simulink model "main_sim_adapt_Gref_SP"  (Simulink 7.2)
settings: Solver=ode2  SolverMode=SingleTasking  StartTime=0.0  StopTime=tsim_max  FixedStep=dtsim  RelTol=1e-3
StopFcn:
  | %mkplt
values from neighbouring files (symbols this model uses):
  aero_surf_qbar_off = get_value('aero_surf_qbar_off')    [setup_claw.m]
  aero_surf_qbar_on = get_value('aero_surf_qbar_on')    [setup_claw.m]
  assertion_time = get_value('assertion_time')    [setup_sim.m]
  att_cmd_select = get_value('att_cmd_select')    [setup_sim.m]
  att_trim_IC = orientation.att'    [setup_claw.m]
  att_type_numbers = cell2mat(struct2cell(att_type))    [setup_constants.m]
  chi_trim_IC = orientation.Vchigam(2)    [setup_claw.m]
  command_time = engage_time + 2.0    [setup_sim.m]
  compute_all_rate_cols = get_value('compute_all_rate_cols')    [setup_claw.m]
  compute_all_vel_cols = get_value('compute_all_vel_cols')    [setup_claw.m]
  da_trim_IC = tmp(1)    [setup_claw.m]
  dc_L2W_IC = orientation.dc_L2W    [setup_claw.m]
  de_trim_IC = tmp(2)    [setup_claw.m]
  dr_trim_IC = tmp(3)    [setup_claw.m]
  dtsim = get_value('dtsim')    [setup_sim.m]
  E_trim_IC = MACH_pos_IC(2)    [setup_claw.m]
  Ed_trim_IC = MACH_vel_IC(2)    [setup_claw.m]
  gain_set = gain_set_next    (= 1)    [setup_claw.m]
  gain_var_struct = rmfield(gain_var_struct,setdiff(fieldnames(gain_var_struct),{'name','size'}))    [setup_claw.m]
  gamma_trim_IC = orientation.Vchigam(3)    [setup_claw.m]
  h_trim_IC = MACH_pos_IC(3)    [setup_claw.m]
  hd_trim_IC = MACH_vel_IC(3)    [setup_claw.m]
  ideal_vel_Kb = MACH_vel_Kb(1)    [setup_sim.m]
  MACH = rmfield(MACH,'vel_throt_lrlim')    [setup_claw.m]
  MACH_att_fb = get_value('MACH_att_fb','onerror',0)    [setup_claw.m]
  MACH_att_int_IC = (1-MACH_att_Kc).*MACH_quat_IC'    [setup_ideal.m]
  MACH_att_Kb = repval(att_kbnom,MACH.att_num_cv)    [setup_claw.m]
  MACH_att_Kc = Ki2Kc(MACH_att_Ki)    [setup_ideal.m]
  MACH_att_Ki = repval(att_fi,MACH.att_num_cv)    [setup_claw.m]
  MACH_gain_mat = vertcat(MACH_gain_mat, this_gain_mat)    [setup_claw.m]
  MACH_mass_IC = obac_params.mass_IC    [setup_claw.m]
  MACH_pos_IC = x_obac_IC(MACH.NEh_idx)    [setup_claw.m]
  MACH_pos_int_IC = (1-MACH_pos_Kc).*MACH_pos_IC' + MACH_vel_IC'./MACH_pos_Kb    [setup_ideal.m]
  MACH_pos_Kb = repval(pos_kbnom,MACH.pos_num_cv)    [setup_claw.m]
  MACH_pos_Kc = Ki2Kc(MACH_pos_Ki)    [setup_ideal.m]
  MACH_pos_Ki = repval(pos_fi,MACH.pos_num_cv)    [setup_claw.m]
  MACH_pqr_Bmat_IC = Bo(MACH.pqr_idx,MACH.pqr_u_idx)    [setup_claw.m]
  MACH_pqr_IC = pqr_trim_IC    [setup_claw.m]
  MACH_pqr_int_IC = (1-MACH_pqr_Kc).*MACH_pqr_IC'    [setup_ideal.m]
  MACH_pqr_Kb = repval(pqr_kbnom,MACH.pqr_num_cv)    [setup_claw.m]
  MACH_pqr_Kc = Ki2Kc(MACH_pqr_Ki)    [setup_ideal.m]
  MACH_pqr_Ki = repval(pqr_fi,MACH.pqr_num_cv)    [setup_claw.m]
  MACH_pqr_u_IC = [ vanes_trim_IC; tvc_trim_IC; rcs_trim_IC ]    [setup_claw.m]
  MACH_quat_IC = quat_trim_IC    [setup_claw.m]
  MACH_throttle_IC = throttle_trim_IC    [setup_claw.m]
  MACH_U_nom_IC = zeros(MACH.num_u,1)    [setup_claw.m]
  MACH_vel_Bmat_IC = MACH_vel_Bmat_IC*inv(vel_perts)    [setup_claw.m]
  MACH_vel_cvdnom_IC = repval(get_value('vel_cvdnom_IC','onerror',MACH_vel_cvdnom_IC),length(MACH_vel_cvdnom_IC))'    [setup_claw.m]
  MACH_vel_IC = orientation.NdEdhd'    [setup_claw.m]
  MACH_vel_int_IC = (1-MACH_vel_Kc).*MACH_vel_IC'    [setup_ideal.m]
  MACH_vel_Kb = repval(vel_kbnom,MACH.vel_num_cv)    [setup_claw.m]
  MACH_vel_Kc = Ki2Kc(MACH_vel_Ki)    [setup_ideal.m]
  MACH_vel_Ki = repval(vel_fi,MACH.vel_num_cv)    [setup_claw.m]
  MACH_vel_uold_IC = [ MACH_quat_IC; MACH_throttle_IC ]    [setup_claw.m]
  N_trim_IC = MACH_pos_IC(1)    [setup_claw.m]
  Nd_trim_IC = MACH_vel_IC(1)    [setup_claw.m]
  obac_params = define_model('obac', get_value('obac_model_type'))    [setup_claw.m]
  pos_cmd_select = get_value('pos_cmd_select')    [setup_sim.m]
  pqr_trim_IC = [ 0 0 0 ]'    [setup_claw.m]
  rate_cmd_select = get_value('rate_cmd_select')    [setup_sim.m]
  rcs_cvddes_thresh = get_value('rcs_cvddes_thresh')    [setup_claw.m]
  reset_camcmd_on_entry = get_value('reset_camcmd_on_entry')    [setup_claw.m]
  throttle_trim_IC = u_obac_IC(MACH.throttle_idx)    [setup_claw.m]
  trac_params = define_model('trac', get_value('trac_model_type','onerror',obac_params.model_type))    [setup_sim.m]
  use_auto_att_type = get_value('use_auto_att_type','onerror',0)    [setup_claw.m]
  use_eow_as_iv = get_value('use_eow_as_iv')    [setup_claw.m]
  use_full_surf_cmd = get_value('use_full_surf_cmd')    [setup_sim.m]
  use_nav = get_value('use_nav')    [setup_claw.m]
  use_NdEdh_pos = get_value('use_NdEdh_pos')    [setup_claw.m]
  use_pos_fltpath_lim = get_value('use_pos_fltpath_lim')    [setup_claw.m]
  use_throt_estimate = get_value('use_throt_estimate')    [setup_claw.m]
  use_variable_mass = get_value('use_variable_mass')    [setup_claw.m]
  use_wind_est = get_value('use_wind_est')    [setup_claw.m]
  V_trim_IC = orientation.Vchigam(1)    [setup_claw.m]
  vel_cmd_ramp_time = get_value('vel_cmd_ramp_time')    [setup_claw.m]
  vel_cmd_select = get_value('vel_cmd_select')    [setup_sim.m]
  x_trac_IC = x_obac_IC    [setup_sim.m]
undefined symbols (not defined in the file or in its folder): accel_cmd, alpha_trim, Am, att_type, B1, bb_ellipsoid, bb_params, Bm, C, constants, cosA, DiscIntNeverNeededParam, DZkx, DZtheta, E_rwy, Ed_cmd, eow_boundary, flag_autoadapt, flag_exsig, flag_uad, full_surf_llim, full_surf_ulim, gam_cmd_descent, gam_cmd_preflare, gamdot_cmd_descent, gamdot_cmd_flare, gamdot_cmd_preflare, Gamtheta, Gamx, hd_cmd, in_error_thresh, in_exsig_vecin, in_exsig_vecout, in_reset_stoptime, in_t_exsig, in_t_timer, in_tadaptoff_forced, in_tadapton_forced, Kb, Kxhat0, Kxnom, Kxstar, max_chi_cmd, max_LOS_rate, max_vel_cmd, min_chi_cmd, min_vel_cmd, modes, N_rwy, Nd_cmd, Nrbf, P, pos, Sig, sinA, target_pos_IC, target_range_blind, target_range_detect, target_range_homing, target_vel_IC ... (+11)
libraries: simulink x44, utility_lib x36, mach_lib x24, model_lib x13, simulink_need_slupdate x8, models x8
(part 2 of 8)

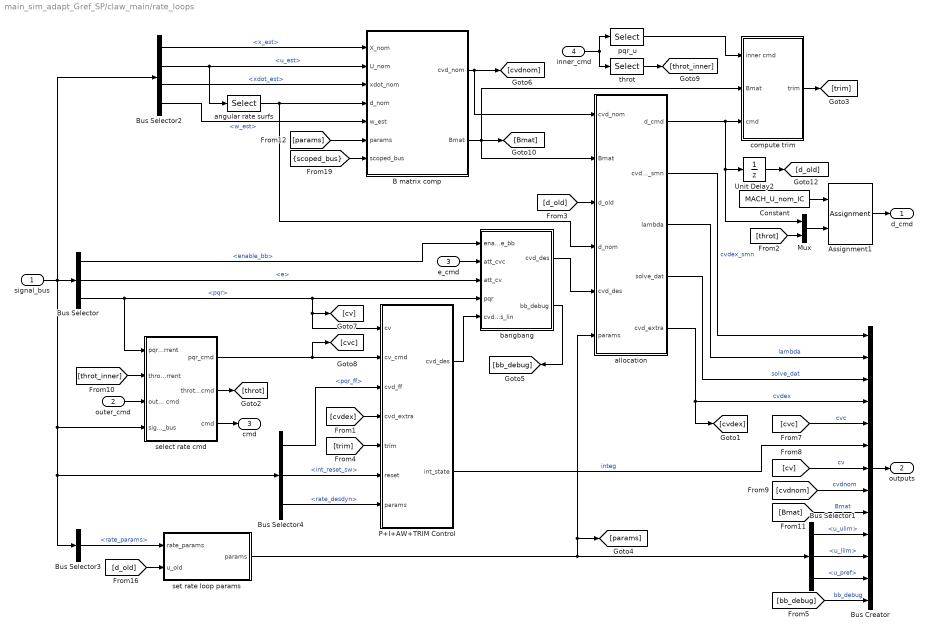
== system main_sim_adapt_Gref_SP/claw_main/rate_loops ==
  signal_bus : Inport  OutDataType=sfix(16)  OutScaling=2^0
  outer_cmd : Inport  Port=2  OutDataType=sfix(16)  OutScaling=2^0
  e_cmd : Inport  Port=3  OutDataType=sfix(16)  OutScaling=2^0
  inner_cmd : Inport  Port=4  OutDataType=sfix(16)  OutScaling=2^0
  Assignment1 : Assignment  IndexOptions=Index vector (dialog)  Indices=[MACH.pqr_u_idx MACH.throttle_idx]  OutputSizes=[1 1]
  B matrix comp : Subsystem  TreatAsAtomicUnit=on
  Bus Creator : BusCreator  Inputs=13
  Bus Selector : BusSelector  OutputSignals=control_params.enable_bb,x_est.e,x_est.pqr
  Bus Selector1 : BusSelector  OutputSignals=u_ulim,u_llim,u_pref
  Bus Selector2 : BusSelector  OutputSignals=x_est,u_est,xdot_est,y_meas.w_est
  Bus Selector3 : BusSelector  OutputSignals=control_params.rate_params
  Bus Selector4 : BusSelector  OutputSignals=feed_forward.pqr_ff,mode_sw.int_reset_sw,control_params.rate_desdyn
  Constant : Constant  Value=MACH_U_nom_IC  OutDataType=sfix(16)  OutScaling=2^0
  Mux : Mux  Inputs=2
  P+I+AW+TRIM Control : Subsystem  AncestorBlock=mach_lib/P+I+AW+TRIM Control
  Unit Delay2 : UnitDelay  X0=MACH_pqr_u_IC  SampleTime=-1
  allocation : Subsystem
  angular rate surfs : Selector  InputPortWidth=MACH.num_u  IndexOptions=Index vector (dialog)  Indices=MACH.pqr_u_idx  OutputSizes=1
  bangbang : Subsystem
  compute trim : Subsystem
  pqr_u : Selector  InputPortWidth=MACH.num_u  IndexOptions=Index vector (dialog)  Indices=MACH.pqr_u_idx  OutputSizes=1
  select rate cmd : Subsystem
  set rate loop params : Subsystem
  throt : Selector  InputPortWidth=MACH.num_u  IndexOptions=Index vector (dialog)  Indices=MACH.throttle_idx  OutputSizes=1
  d_cmd : Outport  OutDataType=sfix(16)  OutScaling=2^0
  outputs : Outport  Port=2  OutDataType=sfix(16)  OutScaling=2^0
  cmd : Outport  Port=3  OutDataType=sfix(16)  OutScaling=2^0
  wires:
  angular rate surfs/1 -> B matrix comp/4(d_nom), allocation/4(d_nom)
  outer_cmd/1 -> select rate cmd/3(outer cmd)
  B matrix comp/1(cvd_nom) -> [cvdnom], allocation/1(cvd_nom)
  P+I+AW+TRIM Control/2(int_state) -> Bus Creator/6  "integ"
  signal_bus/1 -> Bus Selector2/1, Bus Selector/1, Bus Selector3/1, Bus Selector4/1, select rate cmd/4(signal_bus)
  compute trim/1(trim) -> [trim]
  inner_cmd/1 -> pqr_u/1, throt/1
  select rate cmd/2(throt_cmd) -> [throt]
  select rate cmd/1(pqr_cmd) -> [cvc], P+I+AW+TRIM Control/2(cv_cmd)
  [throt_inner] -> select rate cmd/2(throt_current)
  [cvc] -> Bus Creator/5  "cvc"
  [cv] -> Bus Creator/7  "cv"
  [cvdnom] -> Bus Creator/8  "cvdnom"
  set rate loop params/1(params) -> Bus Selector1/1, allocation/6(params), [params]
  Assignment1/1 -> d_cmd/1
  throt/1 -> [throt_inner]
  [trim] -> P+I+AW+TRIM Control/5(trim)
  [cvdex] -> P+I+AW+TRIM Control/4(cvd_extra)
  Bus Selector/3 -> select rate cmd/1(pqr_current), bangbang/4(pqr), P+I+AW+TRIM Control/1(cv), [cv]  "<pqr>"
  Bus Selector4/1 -> P+I+AW+TRIM Control/3(cvd_ff)  "<pqr_ff>"
  Bus Selector4/2 -> P+I+AW+TRIM Control/6(reset)  "<int_reset_sw>"
  [Bmat] -> Bus Creator/9  "Bmat"
  Bus Selector1/1 -> Bus Creator/10  "<u_ulim>"
  Bus Selector1/2 -> Bus Creator/11  "<u_llim>"
  [d_old] -> set rate loop params/2(u_old)
  pqr_u/1 -> compute trim/1(inner cmd)
  Constant/1 -> Assignment1/1
  Mux/1 -> Assignment1/2
  Bus Selector2/1 -> B matrix comp/1(X_nom)  "<x_est>"
  Bus Selector2/2 -> angular rate surfs/1, B matrix comp/2(U_nom)  "<u_est>"
  Bus Selector2/3 -> B matrix comp/3(xdot_nom)  "<xdot_est>"
  Bus Selector2/4 -> B matrix comp/5(w_est)  "<w_est>"
  Bus Selector1/3 -> Bus Creator/12  "<u_pref>"
  allocation/5(cvd_extra) -> Bus Creator/4, [cvdex]  "cvdex"
  [throt] -> Mux/2
  Unit Delay2/1 -> [d_old]
  allocation/1(d_cmd) -> compute trim/3(cmd), Mux/1, Unit Delay2/1
  [d_old] -> allocation/3(d_old)
  B matrix comp/2(Bmat) -> compute trim/2(Bmat), [Bmat], allocation/2(Bmat)
  allocation/3(lambda) -> Bus Creator/2  "lambda"
  allocation/4(solve_dat) -> Bus Creator/3  "solve_dat"
  Bus Creator/1 -> outputs/1
  [scoped_bus] -> B matrix comp/7(scoped_bus)
  [params] -> B matrix comp/6(params)
  Bus Selector4/3 -> P+I+AW+TRIM Control/7(params)  "<rate_desdyn>"
  allocation/2(cvd_extra_smn) -> Bus Creator/1  "cvdex_smn"
  bangbang/1(cvd_des) -> allocation/5(cvd_des)
  e_cmd/1 -> bangbang/2(att_cvc)
  Bus Selector/2 -> bangbang/3(att_cv)  "<e>"
  P+I+AW+TRIM Control/1(cvd_des) -> bangbang/5(cvd_des_lin)
  Bus Selector/1 -> bangbang/1(enable_bb)  "<enable_bb>"
  bangbang/2(bb_debug) -> [bb_debug]
  [bb_debug] -> Bus Creator/13  "bb_debug"
  select rate cmd/3(cmd) -> cmd/1
  Bus Selector3/1 -> set rate loop params/1(rate_params)  "<rate_params>"

== system main_sim_adapt_Gref_SP/claw_main/servo commands  when not engaged ==
  note: for OAV/MAV during "pre-takeoff",
      |  the rate inner_cmd throt was set to takeoff throt
      | to allow integrators to trim for anticipated takeoff.
      | This should be revisited within current CLAW
      | before being used again.
  signal_bus : Inport  OutDataType=sfix(16)  OutScaling=2^0
  outer_cmd : Inport  Port=2  OutDataType=sfix(16)  OutScaling=2^0
  Bus Selector1 : BusSelector  OutputSignals=mode_sw.pre_takeoff_sw,mode_sw.engaged_sw,mode_sw.full_surf_cmd_sw,cmd_bus.autopilot_cmd,full_surf.full_surf_cmd
  Constant1 : Constant  Value=MACH.pre_takeoff_u_backtrim  OutDataType=sfix(16)  OutScaling=2^0
  Multiport Switch : MultiPortSwitch  Inputs=2  zeroidx=on
  Multiport Switch1 : MultiPortSwitch  Inputs=2  zeroidx=on
  Multiport Switch2 : MultiPortSwitch  Inputs=2  zeroidx=on
  pseudo surf cmd : Subsystem
  u_out : Outport  OutDataType=sfix(16)  OutScaling=2^0
  u_backtrim : Outport  Port=2  OutDataType=sfix(16)  OutScaling=2^0
  wires:
  signal_bus/1 -> Bus Selector1/1
  Bus Selector1/1 -> Multiport Switch/1  "<pre_takeoff_sw>"
  Multiport Switch1/1 -> Multiport Switch/2, u_out/1
  Constant1/1 -> Multiport Switch/3
  Bus Selector1/2 -> Multiport Switch1/1  "<engaged_sw>"
  Bus Selector1/3 -> Multiport Switch2/1  "<full_surf_cmd_sw>"
  Bus Selector1/4 -> pseudo surf cmd/1(autopilot_cmd)  "<autopilot_cmd>"
  pseudo surf cmd/1(surf_cmd) -> Multiport Switch2/2
  Bus Selector1/5 -> Multiport Switch2/3  "<full_surf_cmd>"
  Multiport Switch2/1 -> Multiport Switch1/2
  outer_cmd/1 -> Multiport Switch1/3
  Multiport Switch/1 -> u_backtrim/1

== system main_sim_adapt_Gref_SP/claw_main/set scoped signals ==
  signal_bus : Inport  OutDataType=sfix(16)  OutScaling=2^0
  Bus Selector3 : BusSelector  OutputSignals=y_meas.h_geodetic,mode_sw.use_held_aero_obac_sw,y_meas.w_est,y_meas.NEh_dot,mode_sw.att_type,u_est,engines
  Gain1 : Gain  Orientation=left  Gain=use_variable_mass  ParameterDataType=sfix(16)  ParameterScaling=2^0  OutDataType=sfix(16)  OutScaling=2^0
  hold altitude : model_lib/hold input  SystemSampleTime=-1
  mass : DiscreteIntegrator  gainval=1  InitialCondition=MACH_mass_IC  SampleTime=-1  OutDataType=sfix(16)  OutScaling=2^0  ICPrevOutput=DiscIntNeverNeededParam  ICPrevScaledInput=DiscIntNeverNeededParam
  set scoped bus : model_lib/set scoped bus  SystemSampleTime=-1  vehicle_params=obac_params
  set scoped signals : model_lib/set scoped signals  SystemSampleTime=-1
  scoped_bus : Outport  OutDataType=sfix(16)  OutScaling=2^0
  wires:
  signal_bus/1 -> Bus Selector3/1
  Gain1/1 -> mass/1
  Bus Selector3/1 -> hold altitude/1  "<h_geodetic>"
  set scoped bus/2 -> Gain1/1
  set scoped bus/1 -> set scoped signals/1, scoped_bus/1
  mass/1 -> set scoped bus/7
  Bus Selector3/2 -> hold altitude/2  "<use_held_aero_obac_sw>"
  hold altitude/1 -> set scoped bus/1
  Bus Selector3/3 -> set scoped bus/2  "<w_est>"
  Bus Selector3/4 -> set scoped bus/3  "<NEh_dot>"
  Bus Selector3/5 -> set scoped bus/4  "<att_type>"
  Bus Selector3/6 -> set scoped bus/5  "<u_est>"
  Bus Selector3/7 -> set scoped bus/6  "<engines>"

== system main_sim_adapt_Gref_SP/claw_main/state est ==
  u_old : Inport  OutDataType=sfix(16)  OutScaling=2^0
  sensors : Inport  Port=2  OutDataType=sfix(16)  OutScaling=2^0
  signal_bus : Inport  Port=3  OutDataType=sfix(16)  OutScaling=2^0
  Bus Creator : BusCreator  Inputs=12
  Bus Creator1 : BusCreator  Inputs=6
  Bus Selector : BusSelector  OutputSignals=mode_sw.reset_pos_sw,mode_sw.nav_enable_sw,mode_sw.wind_est_sw
  Bus Selector1 : BusSelector  OutputSignals=nav_ok,pqr,NED_dot,latlonh,e
  Bus Selector2 : BusSelector  OutputSignals=aero_env.Mach,aero_env.vel,aero_env.alpha,aero_env.beta,aero_env.uvw_rw,aero_env.qbar
  Bus Selector3 : BusSelector  OutputSignals=u_meas,seeker,accels_cg
  Logical Operator : Logic  AllPortsSameDT=off  OutDataTypeMode=boolean  OutDataTypeStr=boolean
  beta_360 : Fcn  Expr=atan2(u(2),u(1))
  cl model : models/gtm-obac  SystemSampleTime=-1
  process inputs : Subsystem
  process sensors : Subsystem
  wind estimator : Subsystem
  y_meas : Outport  OutDataType=sfix(16)  OutScaling=2^0
  x_est : Outport  Port=2  OutDataType=sfix(16)  OutScaling=2^0
  xdot_est : Outport  Port=3  OutDataType=sfix(16)  OutScaling=2^0
  u_est : Outport  Port=4  OutDataType=sfix(16)  OutScaling=2^0
  aero_env_est : Outport  Port=5  OutDataType=sfix(16)  OutScaling=2^0
  w_est_debug : Outport  Port=6  OutDataType=sfix(16)  OutScaling=2^0
  wires:
  sensors/1 -> Bus Selector3/1, process inputs/2(sensors), wind estimator/3(sensors), Bus Selector1/1
  wind estimator/1(w_est) -> cl model/3, Bus Creator/12  "w_est"
  process sensors/8(dircos) -> wind estimator/1(dircos), Bus Creator/11  "dircos"
  cl model/1 -> xdot_est/1
  process sensors/9(x_est) -> cl model/1, wind estimator/2(x), x_est/1
  signal_bus/1 -> Bus Selector/1
  Bus Selector/1 -> process sensors/1(reset_pos)  "<reset_pos_sw>"
  Bus Selector/3 -> wind estimator/5(wind_est_sw)  "<wind_est_sw>"
  process inputs/1(u_est) -> u_est/1, cl model/2, wind estimator/4(u)
  Bus Selector1/2 -> process sensors/3(pqr)  "<pqr>"
  Bus Selector1/3 -> process sensors/4(NED_dot)  "<NED_dot>"
  Bus Selector1/4 -> process sensors/5(latlonh)  "<latlonh>"
  Bus Selector1/5 -> process sensors/6(e)  "<e>"
  process sensors/2(h_geodetic) -> Bus Creator/5  "h_geodetic"
  process sensors/3(NEh_nav) -> Bus Creator/6  "NEh_nav"
  process sensors/4(nav_valid) -> Bus Creator/7  "nav_valid"
  process sensors/5(NEh_dot) -> Bus Creator/8  "NEh_dot"
  process sensors/1(vehicle_origin) -> Bus Creator/4  "vehicle_origin"
  process sensors/7(cvc_origin) -> Bus Creator/10  "cvc_origin"
  u_old/1 -> process inputs/1(u_old)
  wind estimator/2(w_est_debug) -> w_est_debug/1
  cl model/2 -> Bus Selector2/1
  Bus Creator1/1 -> aero_env_est/1
  Logical Operator/1 -> process sensors/2(nav_ok)
  Bus Selector1/1 -> Logical Operator/2  "<nav_ok>"
  Bus Selector/2 -> Logical Operator/1  "<nav_enable_sw>"
  Bus Selector2/5 -> beta_360/1  "<uvw_rw>"
  process sensors/6(dc_fltpath) -> Bus Creator/9  "dc_fltpath"
  beta_360/1 -> Bus Creator1/5  "beta_360"
  Bus Selector2/1 -> Bus Creator1/1  "<Mach>"
  Bus Selector2/2 -> Bus Creator1/2  "<vel>"
  Bus Selector2/3 -> Bus Creator1/3  "<alpha>"
  Bus Selector2/4 -> Bus Creator1/4  "<beta>"
  Bus Selector2/6 -> Bus Creator1/6  "<qbar>"
  Bus Selector3/1 -> Bus Creator/1  "<u_meas>"
  Bus Selector3/2 -> Bus Creator/2  "<seeker>"
  Bus Selector3/3 -> Bus Creator/3  "<accels_cg>"
  Bus Creator/1 -> y_meas/1

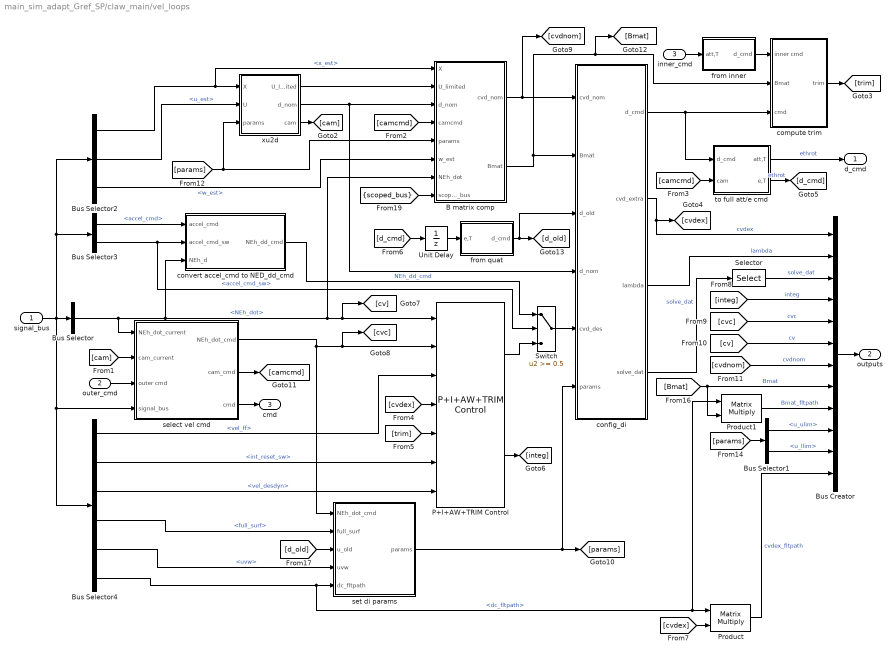
== system main_sim_adapt_Gref_SP/claw_main/vel_loops ==
  signal_bus : Inport  OutDataType=sfix(16)  OutScaling=2^0
  outer_cmd : Inport  Port=2  OutDataType=sfix(16)  OutScaling=2^0
  inner_cmd : Inport  Port=3  OutDataType=sfix(16)  OutScaling=2^0
  B matrix comp : Subsystem
  Bus Creator : BusCreator  Inputs=12
  Bus Selector : BusSelector  OutputSignals=y_meas.NEh_dot
  Bus Selector1 : BusSelector  OutputSignals=u_ulim,u_llim
  Bus Selector2 : BusSelector  OutputSignals=x_est,u_est,y_meas.w_est
  Bus Selector3 : BusSelector  OutputSignals=control_params.accel_cmd,control_params.accel_cmd_sw
  Bus Selector4 : BusSelector  OutputSignals=feed_forward.vel_ff,mode_sw.int_reset_sw,control_params.vel_desdyn,full_surf,x_est.uvw,y_meas.dc_fltpath
  P+I+AW+TRIM Control : mach_lib/P+I+AW+TRIM Control  SystemSampleTime=-1
  Product : Product  Multiplication=Matrix(*)  OutDataType=sfix(16)  OutScaling=2^0  RndMeth=Zero
  Product1 : Product  Multiplication=Matrix(*)  OutDataType=sfix(16)  OutScaling=2^0  RndMeth=Zero
  Selector : Selector  NumberOfDimensions=2  InputPortWidth=MACH.num_u  IndexOptions=Index vector (dialog),Index vector (dialog)  Indices=1:9,1:2  OutputSizes=1
  Switch : Switch  Threshold=0.5
  Unit Delay : UnitDelay  X0=MACH_vel_uold_IC  SampleTime=-1
  compute trim : Subsystem
  config_di : Subsystem  BlockChoice=di_smn  mask{num_cv=MACH.vel_num_cv, num_u=MACH.vel_num_u, wght_cv_type=MACH.vel_wght_cv_type}
      link override di_smn/config_smn/smn_sfunc: sfunc_name=MACH.smn_sfunc_name
      link override di_smn/config_smn/smn_sfunc/S-Function: FunctionName=smn_sfunc_gam_mpass_epsposdef
      settings: AttributesFormatString=%<BlockChoice>  TemplateBlock=mach_lib/config_di  MemberBlocks=di_pseudoinv,di_smn
  convert accel_cmd to NED_dd_cmd : Subsystem  TreatAsAtomicUnit=on
  from inner : Subsystem
  from quat : Subsystem
  select vel cmd : Subsystem
  set di params : Subsystem
  to full att/e cmd : Subsystem
  xu2d : Subsystem
  d_cmd : Outport  OutDataType=sfix(16)  OutScaling=2^0
  outputs : Outport  Port=2  OutDataType=sfix(16)  OutScaling=2^0
  cmd : Outport  Port=3  OutDataType=sfix(16)  OutScaling=2^0
  wires:
  B matrix comp/2(Bmat) -> config_di/2(Bmat), compute trim/2(Bmat), [Bmat]
  to full att/e cmd/1(att,T) -> d_cmd/1  "ethrot"
  config_di/1(d_cmd) -> compute trim/3(cmd), to full att/e cmd/1(d_cmd)
  P+I+AW+TRIM Control/2 -> [integ]
  xu2d/2(d_nom) -> config_di/4(d_nom), B matrix comp/3(d_nom)
  Bus Selector/1 -> convert accel_cmd to NED_dd_cmd/3(NEh_d), B matrix comp/7(NEh_dot), P+I+AW+TRIM Control/1, [cv], select vel cmd/1(NEh_dot_current)  "<NEh_dot>"
  xu2d/3(cam) -> [cam]
  [cam] -> select vel cmd/2(cam_current)
  compute trim/1(trim) -> [trim]
  inner_cmd/1 -> from inner/1(att,T)
  from inner/1(d_cmd) -> compute trim/1(inner cmd)
  [camcmd] -> to full att/e cmd/2(cam)
  Bus Selector2/3 -> B matrix comp/6(w_est)  "<w_est>"
  [d_cmd] -> Unit Delay/1
  Unit Delay/1 -> from quat/1(e,T)
  set di params/1(params) -> [params], config_di/6(params)
  [params] -> xu2d/3(params), B matrix comp/5(params)
  xu2d/1(U_limited) -> B matrix comp/2(U_limited)
  [integ] -> Bus Creator/4  "integ"
  [cvc] -> Bus Creator/5  "cvc"
  [cv] -> Bus Creator/6  "cv"
  [cvdnom] -> Bus Creator/7  "cvdnom"
  [trim] -> P+I+AW+TRIM Control/5
  [cvdex] -> P+I+AW+TRIM Control/4
  Bus Selector4/2 -> P+I+AW+TRIM Control/6  "<int_reset_sw>"
  Bus Selector4/1 -> P+I+AW+TRIM Control/3  "<vel_ff>"
  B matrix comp/1(cvd_nom) -> [cvdnom], config_di/1(cvd_nom)
  [Bmat] -> Product1/2, Bus Creator/8  "Bmat"
  config_di/2(cvd_extra) -> [cvdex], Bus Creator/1  "cvdex"
  from quat/1(d_cmd) -> [d_old], config_di/3(d_old)
  Bus Selector4/4 -> set di params/2(full_surf)  "<full_surf>"
  Product/1 -> Bus Creator/12  "cvdex_fltpath"
  [params] -> Bus Selector1/1
  Bus Selector1/1 -> Bus Creator/10  "<u_ulim>"
  Bus Selector1/2 -> Bus Creator/11  "<u_llim>"
  [d_old] -> set di params/3(u_old)
  Bus Selector4/5 -> set di params/4(uvw)  "<uvw>"
  config_di/3(lambda) -> Bus Creator/2  "lambda"
  config_di/4(solve_dat) -> Selector/1  "solve_dat"
  [cvdex] -> Product/2
  Selector/1 -> Bus Creator/3  "solve_dat"
  [camcmd] -> B matrix comp/4(camcmd)
  [scoped_bus] -> B matrix comp/8(scoped_bus)
  Bus Selector2/1 -> xu2d/1(X), B matrix comp/1(X)  "<x_est>"
  Bus Selector2/2 -> xu2d/2(U)  "<u_est>"
  Bus Selector4/3 -> P+I+AW+TRIM Control/7  "<vel_desdyn>"
  Bus Selector3/1 -> convert accel_cmd to NED_dd_cmd/1(accel_cmd)  "<accel_cmd>"
  Switch/1 -> config_di/5(cvd_des)
  P+I+AW+TRIM Control/1 -> Switch/3
  convert accel_cmd to NED_dd_cmd/1(NEh_dd_cmd) -> Switch/1  "NEh_dd_cmd"
  signal_bus/1 -> Bus Selector/1, Bus Selector3/1, Bus Selector2/1, Bus Selector4/1, select vel cmd/4(signal_bus)
  Bus Selector3/2 -> convert accel_cmd to NED_dd_cmd/2(accel_cmd_sw), Switch/2  "<accel_cmd_sw>"
  Product1/1 -> Bus Creator/9  "Bmat_fltpath"
  Bus Selector4/6 -> Product/1, Product1/1, set di params/5(dc_fltpath)  "<dc_fltpath>"
  to full att/e cmd/2(e,T) -> [d_cmd]  "ethrot"
  outer_cmd/1 -> select vel cmd/3(outer cmd)
  select vel cmd/3(cmd) -> cmd/1
  select vel cmd/2(cam_cmd) -> [camcmd]
  select vel cmd/1(NEh_dot_cmd) -> set di params/1(NEh_dot_cmd), P+I+AW+TRIM Control/2, [cvc]
  Bus Creator/1 -> outputs/1

== system main_sim_adapt_Gref_SP/control input (modified)/Add Excitation ==
  In : Inport
  Adapt On-Off : Inport  Port=2
  Bus Selector1 : BusSelector  OutputSignals=command
  CMD : Scope
      settings: TimeRange=25  YMin=0  YMax=2  SaveName=ScopeData20
  CMD + EXC : Scope
      settings: TimeRange=25  YMin=-1  YMax=15  SaveName=ScopeData8
  Demux : Demux  Outputs=[1 1 1 1]
  EXC : Scope
      settings: TimeRange=25  YMin=-2  YMax=2  SaveName=ScopeData23
  Excitation  Signal : Subsystem
  Gain1 : Gain  Gain=180/pi  ParameterDataType=sfix(16)  ParameterScaling=2^0  OutDataType=sfix(16)  OutScaling=2^0
  Gain2 : Gain  Gain=180/pi  ParameterDataType=sfix(16)  ParameterScaling=2^0  OutDataType=sfix(16)  OutScaling=2^0
  Gain3 : Gain  Gain=180/pi  ParameterDataType=sfix(16)  ParameterScaling=2^0  OutDataType=sfix(16)  OutScaling=2^0
  Mux : Mux
  Step : Step  Time=in_t_exsig  SampleTime=MACH.dt
  Sum : Sum  Inputs=|++  OutDataType=sfix(16)  OutScaling=2^0
  Terminator : Terminator
  Unit Delay : UnitDelay  SampleTime=MACH.dt
  Out : Outport
  wires:
  Mux/1 -> Out/1
  In/1 -> Bus Selector1/1
  Demux/4 -> Mux/4
  Excitation  Signal/1(exsig) -> Sum/2, Gain3/1
  Sum/1 -> Mux/2, Gain2/1
  Demux/2 -> Sum/1, Gain1/1
  Demux/3 -> Mux/3
  Demux/1 -> Mux/1
  Bus Selector1/1 -> Demux/1  "<command>"
  Gain2/1 -> CMD + EXC/1
  Gain1/1 -> CMD/1
  Gain3/1 -> EXC/1
  Step/1 -> Terminator/1
  Adapt On-Off/1 -> Unit Delay/1
  Unit Delay/1 -> Excitation  Signal/Enable

== system main_sim_adapt_Gref_SP/control input (modified)/control input ==
  Rate Transition1 : RateTransition  OutPortSampleTime=MACH.dt
  form control input : Subsystem  SystemSampleTime=MACH.dt
  generate commands : Subsystem
  control_input : Outport  OutDataType=sfix(16)  OutScaling=2^0
  wires:
  generate commands/1(cmd_bus) -> form control input/1(cmd_bus)
  form control input/1(control_input) -> Rate Transition1/1
  Rate Transition1/1 -> control_input/1

== system main_sim_adapt_Gref_SP/control input (modified)/ideal responses ==
  control_input : Inport  OutDataType=sfix(16)  OutScaling=2^0
      settings: BusObject=control_input_bus
  ideal att rate response : Subsystem
  ideal pos vel response : Subsystem
  wires:
  control_input/1 -> ideal pos vel response/1(control_input), ideal att rate response/1(control_input)

== system main_sim_adapt_Gref_SP/vehicle_model/a/c model ==
  u : Inport  OutDataType=sfix(16)  OutScaling=2^0
  integrate_state : Inport  Port=2  OutDataType=sfix(16)  OutScaling=2^0
  NED_wind : Inport  Port=3  OutDataType=sfix(16)  OutScaling=2^0
  Logical Operator : Logic  Operator=NOT  AllPortsSameDT=off  OutDataTypeMode=boolean  OutDataTypeStr=boolean
  Product : Product  OutDataType=sfix(16)  OutScaling=2^0  RndMeth=Zero
  e mag error feedback : model_lib/e mag error feedback  SystemSampleTime=-1
  vehicle model : models/gtm-trac  SystemSampleTime=-1  vehicle_params=trac_params
  vehicle state integrator : Integrator  ExternalReset=level  InitialCondition=x_trac_IC
  x : Outport  OutDataType=sfix(16)  OutScaling=2^0
  xdot : Outport  Port=2  OutDataType=sfix(16)  OutScaling=2^0
  y : Outport  Port=3  OutDataType=sfix(16)  OutScaling=2^0
  wires:
  u/1 -> vehicle model/2
  vehicle state integrator/1 -> x/1, vehicle model/1, e mag error feedback/1
  integrate_state/1 -> Logical Operator/1, Product/2
  Product/1 -> xdot/1, vehicle state integrator/1
  Logical Operator/1 -> vehicle state integrator/2
  NED_wind/1 -> vehicle model/3
  vehicle model/2 -> y/1
  e mag error feedback/1 -> Product/1
  vehicle model/1 -> e mag error feedback/2

== system main_sim_adapt_Gref_SP/vehicle_model/apply additional limits ==
  effector_limits_in : Inport  OutDataType=sfix(16)  OutScaling=2^0
  Bus Assignment : BusAssignment  AssignedSignals=u_ulim,u_llim
  Bus Selector : BusSelector  OutputSignals=u_ulim,u_llim
  throt out of fuel limits : model_lib/throt out of fuel limits  SystemSampleTime=-1
  effector_limits : Outport  OutDataType=sfix(16)  OutScaling=2^0
  wires:
  effector_limits_in/1 -> Bus Assignment/1, Bus Selector/1
  Bus Selector/1 -> throt out of fuel limits/1  "<u_ulim>"
  Bus Selector/2 -> throt out of fuel limits/2  "<u_llim>"
  Bus Assignment/1 -> effector_limits/1
  throt out of fuel limits/1 -> Bus Assignment/2
  throt out of fuel limits/2 -> Bus Assignment/3

== system main_sim_adapt_Gref_SP/vehicle_model/set scoped signals ==
  note: Note: att_type is not actually
      | used by the trac
  output_bus : Inport  OutDataType=sfix(16)  OutScaling=2^0
  Bus Selector1 : BusSelector  OutputSignals=x,use_held_aero_trac_sw,NED_wind,xdot,u_servo,engines
  Constant2 : Constant  Value=MACH.att_type  OutDataType=sfix(16)  OutScaling=2^0
  Gain1 : Gain  Orientation=left  Gain=use_variable_mass  ParameterDataType=sfix(16)  ParameterScaling=2^0  OutDataType=sfix(16)  OutScaling=2^0
  NEh_dot : Selector  InputPortWidth=trac_params.num_x  IndexOptions=Index vector (dialog)  Indices=MACH.NEh_idx  OutputSizes=1
  h : Selector  InputPortWidth=MACH.num_x  IndexOptions=Index vector (dialog)  Indices=MACH.NEh_idx(3)  OutputSizes=1
  hold altitude : model_lib/hold input  SystemSampleTime=-1
  mass integrator : Integrator  InitialCondition=trac_params.mass_IC
  set scoped bus : model_lib/set scoped bus  SystemSampleTime=-1  vehicle_params=trac_params
  set scoped signals : model_lib/set scoped signals  SystemSampleTime=-1
  scoped_bus : Outport  OutDataType=sfix(16)  OutScaling=2^0
  wires:
  Bus Selector1/1 -> h/1  "<x>"
  NEh_dot/1 -> set scoped bus/3
  Bus Selector1/3 -> set scoped bus/2  "<NED_wind>"
  Bus Selector1/5 -> set scoped bus/5  "<u_servo>"
  mass integrator/1 -> set scoped bus/7
  set scoped bus/2 -> Gain1/1
  Gain1/1 -> mass integrator/1
  hold altitude/1 -> set scoped bus/1
  h/1 -> hold altitude/1
  Bus Selector1/2 -> hold altitude/2  "<use_held_aero_trac_sw>"
  set scoped bus/1 -> set scoped signals/1, scoped_bus/1
  Constant2/1 -> set scoped bus/4
  Bus Selector1/4 -> NEh_dot/1  "<xdot>"
  output_bus/1 -> Bus Selector1/1
  Bus Selector1/6 -> set scoped bus/6  "<engines>"

== system main_sim_adapt_Gref_SP/vehicle_model/target/seeker model ==
  output_bus : Inport  OutDataType=sfix(16)  OutScaling=2^0
  Bus Selector : BusSelector  OutputSignals=x,xdot
  Bus Selector1 : BusSelector  OutputSignals=LOS_rate,aux_info.azimuth,aux_info.elevation,aux_info.Rground,aux_info.Rslant
  Constant2 : Constant  Value=target_vel_IC  OutDataType=sfix(16)  OutScaling=2^0
  NEh : Selector  InputPortWidth=MACH.num_x  IndexOptions=Index vector (dialog)  Indices=MACH.NEh_idx  OutputSizes=1
  NEh_dot : Selector  InputPortWidth=MACH.num_x  IndexOptions=Index vector (dialog)  Indices=MACH.NEh_idx  OutputSizes=1
  seeker model : Subsystem
  seeker scope : Scope  NumInputPorts=5
      settings: YMin=-1.75~-3.5~-1.75~0~0  YMax=0.25~0.5~0~450000~550000
  target position integrator : Integrator  InitialCondition=target_pos_IC
  seeker : Outport  OutDataType=sfix(16)  OutScaling=2^0
  wires:
  Constant2/1 -> target position integrator/1, seeker model/2(NEh_d_target)
  target position integrator/1 -> seeker model/1(NEh_target)
  NEh/1 -> seeker model/3(NEh)
  NEh_dot/1 -> seeker model/4(NEh_d)
  seeker model/1(seeker) -> seeker/1, Bus Selector1/1
  output_bus/1 -> Bus Selector/1
  Bus Selector/1 -> NEh/1  "<x>"
  Bus Selector/2 -> NEh_dot/1  "<xdot>"
  Bus Selector1/2 -> seeker scope/2  "<azimuth>"
  Bus Selector1/3 -> seeker scope/3  "<elevation>"
  Bus Selector1/4 -> seeker scope/4  "<Rground>"
  Bus Selector1/5 -> seeker scope/5  "<Rslant>"
  Bus Selector1/1 -> seeker scope/1  "<LOS_rate>"

== system main_sim_adapt_Gref_SP/MRAC/Enable Adaptation/Resettable Switch (On with rising signal/ Off with timer) ==
  note: Logic: Internally reset
      | is ready whenevr
      | the switch is off
  In1 : Inport
  reset : Inport  Port=2
  Add : Sum  OutDataType=sfix(16)  OutScaling=2^-10
  Integrator : Integrator  ExternalReset=falling
  Logical Operator : Logic  Orientation=up  Operator=NOT  AllPortsSameDT=off  OutDataTypeMode=boolean  OutDataTypeStr=boolean
  Logical Operator1 : Logic  Orientation=down  Operator=NOT  AllPortsSameDT=off  OutDataTypeMode=boolean  OutDataTypeStr=boolean
  One-time Switch On (With Rising Signal) 1 : Subsystem
  One-time Switch On (With Rising Signal) 2 : Subsystem
  Product : Product  OutDataType=sfix(16)  OutScaling=2^0  RndMeth=Zero
  Relational Operator : RelationalOperator  Operator=>  LogicOutDataTypeMode=boolean  OutDataTypeStr=boolean
  Scope : Scope
      settings: TimeRange=1.5  YMin=0  YMax=2  SaveName=ScopeData8
  Timer : Constant  Value=in_t_timer  OutDataType=sfix(16)  OutScaling=2^0
  Unit Delay Resettable : simulink/Additional Math & Discrete/Additional Discrete/Unit Delay Resettable  Orientation=left  SystemSampleTime=-1  vinit=0.0  tsamp=-1
  Out1 : Outport
  reset ready : Outport  Port=2
  wires:
  Product/1 -> Out1/1, Logical Operator1/1
  In1/1 -> One-time Switch On (With Rising Signal) 1/1(In1)
  One-time Switch On (With Rising Signal) 2/1(Out1) -> Logical Operator/1, Unit Delay Resettable/1
  Timer/1 -> Relational Operator/2
  Relational Operator/1 -> One-time Switch On (With Rising Signal) 2/1(In1), Scope/1
  Integrator/1 -> Relational Operator/1
  One-time Switch On (With Rising Signal) 1/1(Out1) -> Integrator/1, Product/1
  reset/1 -> One-time Switch On (With Rising Signal) 1/2(In2), Unit Delay Resettable/2, One-time Switch On (With Rising Signal) 2/2(In2), Add/1
  Add/1 -> Integrator/2
  Unit Delay Resettable/1 -> Add/2
  Logical Operator/1 -> Product/2
  Logical Operator1/1 -> reset ready/1

== system main_sim_adapt_Gref_SP/claw_main/att_loops/P+I+AW+TRIM Control ==
  cv : Inport  OutDataType=sfix(16)  OutScaling=2^0
  cv cmd : Inport  Port=2  OutDataType=sfix(16)  OutScaling=2^0
  cvd ff : Inport  Port=3  OutDataType=sfix(16)  OutScaling=2^0
  cvdot extra : Inport  Port=4  OutDataType=sfix(16)  OutScaling=2^0
  trim : Inport  Port=5  OutDataType=sfix(16)  OutScaling=2^0
  reset : Inport  Port=6  OutDataType=sfix(16)  OutScaling=2^0
  x0 : Inport  Port=7  OutDataType=sfix(16)  OutScaling=2^0
  Dot Product2 : simulink/Math Operations/Dot Product  InputSameDT=on  OutDataType=sfix(16)  OutScaling=2^-10  DoSatur=off
  P+I+AW+TRIM Control : mach_lib/P+I+AW+TRIM Control  SystemSampleTime=-1
  Product2 : Product  OutDataType=sfix(16)  OutScaling=2^0  SaturateOnIntegerOverflow=on  InputSameDT=on  OutDataTypeStr=Inherit: Same as first input
  Sum : Sum  Inputs=-+|  OutDataType=sfix(16)  OutScaling=2^0  SaturateOnIntegerOverflow=on
  Unit Delay1 : UnitDelay  SampleTime=-1
  fe : Gain  Gain=MACH.att_fe  ParameterDataType=sfix(16)  ParameterScaling=2^0  OutDataType=sfix(16)  OutScaling=2^0  SaturateOnIntegerOverflow=on  OutDataTypeStr=Inherit: Same as input  ParamDataTypeStr=Inherit: Same as input
  cvdot des : Outport  OutDataType=sfix(16)  OutScaling=2^0
  int state : Outport  Port=2  OutDataType=sfix(16)  OutScaling=2^0
  wires:
  cvd ff/1 -> P+I+AW+TRIM Control/3
  cvdot extra/1 -> P+I+AW+TRIM Control/4
  Sum/1 -> P+I+AW+TRIM Control/5
  reset/1 -> P+I+AW+TRIM Control/6
  x0/1 -> P+I+AW+TRIM Control/7
  fe/1 -> Sum/1
  trim/1 -> Sum/2
  Product2/1 -> fe/1
  Unit Delay1/1 -> Dot Product2/2
  Dot Product2/1 -> Product2/2
  P+I+AW+TRIM Control/2 -> int state/1
  P+I+AW+TRIM Control/1 -> Unit Delay1/1, cvdot des/1
  cv cmd/1 -> P+I+AW+TRIM Control/2
  cv/1 -> Product2/1, Dot Product2/1, P+I+AW+TRIM Control/1

== system main_sim_adapt_Gref_SP/claw_main/att_loops/compute trim ==
  inner cmd : Inport  OutDataType=sfix(16)  OutScaling=2^0
  Bmat : Inport  Port=2  OutDataType=sfix(16)  OutScaling=2^0
  cmd : Inport  Port=3  OutDataType=sfix(16)  OutScaling=2^0
  Product : Product  Multiplication=Matrix(*)  OutDataType=sfix(16)  OutScaling=2^0  SaturateOnIntegerOverflow=on  OutDataTypeStr=Inherit: Same as first input
  Sum1 : Sum  Inputs=|+-  OutDataType=sfix(16)  OutScaling=2^0  SaturateOnIntegerOverflow=on
  trim : Outport  OutDataType=sfix(16)  OutScaling=2^0
  wires:
  Product/1 -> trim/1
  Bmat/1 -> Product/1
  Sum1/1 -> Product/2
  inner cmd/1 -> Sum1/1
  cmd/1 -> Sum1/2

== system main_sim_adapt_Gref_SP/claw_main/att_loops/dyn inv ==
  limit_pqr_cmd : Inport  OutDataType=sfix(16)  OutScaling=2^0
  uvw : Inport  Port=2  OutDataType=sfix(16)  OutScaling=2^0
  e nom : Inport  Port=3  OutDataType=sfix(16)  OutScaling=2^0
  e dot des : Inport  Port=4  OutDataType=sfix(16)  OutScaling=2^0
  Dot Product : simulink/Math Operations/Dot Product  InputSameDT=on  OutDataType=sfix(16)  OutScaling=2^-10  DoSatur=off
  Gain4 : Gain  Gain=0.5  ParameterDataType=sfix(16)  ParameterScaling=2^0  OutDataType=sfix(16)  OutScaling=2^0
  Limit rate cmd : Subsystem
  Product4 : Product  OutDataType=sfix(16)  OutScaling=2^0  SaturateOnIntegerOverflow=on  InputSameDT=on  OutDataTypeStr=Inherit: Same as first input
  Product5 : Product  Inputs=**  Multiplication=Matrix(*)  OutDataType=sfix(16)  OutScaling=2^0  SaturateOnIntegerOverflow=on  InputSameDT=on  OutDataTypeStr=Inherit: Same as first input
  Sum4 : Sum  Inputs=++-  OutDataType=sfix(16)  OutScaling=2^0  SaturateOnIntegerOverflow=on  InputSameDT=on  OutDataTypeStr=Inherit: Same as first input
  getedinv : utility_lib/getedinv  SystemSampleTime=-1
  Bmat : Outport  OutDataType=sfix(16)  OutScaling=2^0
  pqr : Outport  Port=2  OutDataType=sfix(16)  OutScaling=2^0
  cvdex : Outport  Port=3  OutDataType=sfix(16)  OutScaling=2^0
  wires:
  Limit rate cmd/1(pqr_limited) -> pqr/1, Product5/2
  Sum4/1 -> cvdex/1
  Product4/1 -> Sum4/2
  Product5/1 -> Sum4/1
  e dot des/1 -> Dot Product/2, Sum4/3, getedinv/1
  e nom/1 -> Product4/1, Dot Product/1, getedinv/2
  Dot Product/1 -> Product4/2
  getedinv/2 -> Gain4/1
  uvw/1 -> Limit rate cmd/2(uvw)
  getedinv/1 -> Limit rate cmd/3(pqr)
  limit_pqr_cmd/1 -> Limit rate cmd/1(limit_pqr_cmd)
  Gain4/1 -> Product5/1, Bmat/1

== system main_sim_adapt_Gref_SP/claw_main/att_loops/low pass filter ==
  e_cmd : Inport  OutDataType=sfix(16)  OutScaling=2^0
  signal_bus : Inport  Port=2  OutDataType=sfix(16)  OutScaling=2^0
  att_ff : Inport  Port=3  OutDataType=sfix(16)  OutScaling=2^0
  Bus Selector4 : BusSelector  OutputSignals=control_params.att_desdyn.kf,control_params.att_desdyn.kb
  Compare To Zero : simulink/Logic and Bit Operations/Compare To Zero  SystemSampleTime=-1  relop===  LogicOutDataTypeMode=boolean  ZeroCross=off
  Constant : Constant  Value=MACH_att_fb  OutDataType=sfix(16)  OutScaling=2^0
  Discrete-Time Integrator : DiscreteIntegrator  ExternalReset=sampled level  InitialConditionSource=external  SampleTime=-1  OutDataType=sfix(16)  OutScaling=2^0  ICPrevOutput=DiscIntNeverNeededParam  ICPrevScaledInput=DiscIntNeverNeededParam
  Product : Product  Inputs=3  OutDataType=sfix(16)  OutScaling=2^0  RndMeth=Zero
  Product1 : Product  OutDataType=sfix(16)  OutScaling=2^0  RndMeth=Zero
  Product2 : Product  OutDataType=sfix(16)  OutScaling=2^0  RndMeth=Zero
  Sum : Sum  Inputs=|+-  OutDataType=sfix(16)  OutScaling=2^0
  Sum1 : Sum  Inputs=++|  OutDataType=sfix(16)  OutScaling=2^0
  cv cmd : Outport  OutDataType=sfix(16)  OutScaling=2^0
  cvd ff : Outport  Port=2  OutDataType=sfix(16)  OutScaling=2^0
  wires:
  Product/1 -> Sum1/2
  e_cmd/1 -> Sum/1, Discrete-Time Integrator/3
  Sum/1 -> Product/3
  Sum1/1 -> Discrete-Time Integrator/1, cvd ff/1
  Discrete-Time Integrator/1 -> Sum/2, cv cmd/1
  signal_bus/1 -> Bus Selector4/1
  att_ff/1 -> Product1/1
  Product1/1 -> Sum1/1
  Compare To Zero/1 -> Discrete-Time Integrator/2
  Bus Selector4/2 -> Product/2  "<kb>"
  Product2/1 -> Product/1, Compare To Zero/1
  Bus Selector4/1 -> Product2/2, Product1/2  "<kf>"
  Constant/1 -> Product2/1

== system main_sim_adapt_Gref_SP/claw_main/att_loops/select att cmd ==
  e_current : Inport  OutDataType=sfix(16)  OutScaling=2^0
  throt_current : Inport  Port=2  OutDataType=sfix(16)  OutScaling=2^0
  outer cmd : Inport  Port=3  OutDataType=sfix(16)  OutScaling=2^0
  signal_bus : Inport  Port=4  OutDataType=sfix(16)  OutScaling=2^0
  Bus Selector1 : BusSelector  OutputSignals=cmd_bus.select_cmd.att
  Compare To Zero : simulink/Logic and Bit Operations/Compare To Zero  SystemSampleTime=-1  relop===  LogicOutDataTypeMode=boolean  ZeroCross=off
  Demux : Demux  Outputs=[ 4 1 ]
  Demux1 : Demux  Outputs=[ 3 MACH.num_u_throt ]
  Demux2 : Demux  Outputs=[ 1 3 ]
  Mux1 : Mux  Inputs=2
  Switch : Switch  Threshold=0.5
  Unit Delay2 : UnitDelay  X0=MACH_throttle_IC  SampleTime=-1
  att2e_ref : utility_lib/att2e_ref  SystemSampleTime=-1
  e2att : utility_lib/e2att  SystemSampleTime=-1
  get direct cmd : Subsystem
  switch att cmd : MultiPortSwitch  zeroidx=on  SaturateOnIntegerOverflow=on
  switch throt cmd : MultiPortSwitch  zeroidx=on  SaturateOnIntegerOverflow=on
  e_cmd : Outport  OutDataType=sfix(16)  OutScaling=2^0
  throt_cmd : Outport  Port=2  OutDataType=sfix(16)  OutScaling=2^0
  cmd : Outport  Port=3  OutDataType=sfix(16)  OutScaling=2^0
  wires:
  switch att cmd/1 -> att2e_ref/1, Mux1/1
  Bus Selector1/1 -> Demux/1  "<att>"
  get direct cmd/2(throt) -> switch throt cmd/3
  throt_current/1 -> Unit Delay2/1
  Demux/2 -> switch throt cmd/1
  outer cmd/1 -> Demux1/1
  Demux1/2 -> switch throt cmd/4
  switch throt cmd/1 -> throt_cmd/1, Mux1/2
  signal_bus/1 -> get direct cmd/1(signal_bus), Bus Selector1/1
  Demux/1 -> Demux2/1
  e_current/1 -> e2att/1, Switch/1, att2e_ref/2
  Unit Delay2/1 -> switch throt cmd/2
  get direct cmd/1(att) -> switch att cmd/3
  e2att/1 -> switch att cmd/2
  Demux1/1 -> switch att cmd/4
  att2e_ref/1 -> Switch/3
  Switch/1 -> e_cmd/1
  Demux2/1 -> Compare To Zero/1
  Demux2/2 -> switch att cmd/1
  Compare To Zero/1 -> Switch/2
  Mux1/1 -> cmd/1

== system main_sim_adapt_Gref_SP/claw_main/grab ExportedGlobal/grab cv variables ==
  In1 : Inport  OutDataType=sfix(16)  OutScaling=2^0
  Bus Selector6 : BusSelector  OutputSignals=rate.cv,att.cv,vel.cv,pos.cv
  Demux1 : Demux  Outputs=3
  Demux2 : Demux
  Demux3 : Demux  Outputs=3
  Demux4 : Demux  Outputs=3
  Mux : Mux  Inputs=13
  Subsystem : Subsystem  TreatAsAtomicUnit=on
      settings: RTWSystemCode=Inline
  Out1 : Outport  OutDataType=sfix(16)  OutScaling=2^0
  wires:
  Subsystem/1(Out1) -> Mux/1  "CLAW_p_cv"
  Subsystem/2(Out2) -> Mux/2  "CLAW_q_cv"
  Subsystem/3(Out3) -> Mux/3  "CLAW_r_cv"
  Subsystem/4(Out4) -> Mux/4  "CLAW_e0_cv"
  Subsystem/5(Out5) -> Mux/5  "CLAW_e1_cv"
  Subsystem/6(Out6) -> Mux/6  "CLAW_e2_cv"
  Subsystem/8(Out8) -> Mux/8  "CLAW_Ndot_cv"
  Subsystem/9(Out9) -> Mux/9  "CLAW_Edot_cv"
  Subsystem/10(Out10) -> Mux/10  "CLAW_hdot_cv"
  Subsystem/11(Out11) -> Mux/11  "CLAW_N_cv"
  Subsystem/12(Out12) -> Mux/12  "CLAW_E_cv"
  Subsystem/13(Out13) -> Mux/13  "CLAW_h_cv"
  Subsystem/7(Out7) -> Mux/7  "CLAW_e3_cv"
  In1/1 -> Bus Selector6/1
  Mux/1 -> Out1/1
  Demux1/1 -> Subsystem/1(In1)
  Demux1/2 -> Subsystem/2(In2)
  Demux1/3 -> Subsystem/3(In3)
  Demux2/1 -> Subsystem/4(In4)
  Demux2/2 -> Subsystem/5(In5)
  Demux2/3 -> Subsystem/6(In6)
  Demux2/4 -> Subsystem/7(In7)
  Demux3/1 -> Subsystem/8(In8)
  Demux3/2 -> Subsystem/9(In9)
  Demux3/3 -> Subsystem/10(In10)
  Demux4/1 -> Subsystem/11(In11)
  Demux4/2 -> Subsystem/12(In12)
  Demux4/3 -> Subsystem/13(In13)
  Bus Selector6/1 -> Demux1/1  "<cv>"
  Bus Selector6/2 -> Demux2/1  "<cv>"
  Bus Selector6/3 -> Demux3/1  "<cv>"
  Bus Selector6/4 -> Demux4/1  "<cv>"

== system main_sim_adapt_Gref_SP/claw_main/grab ExportedGlobal/grab cvcmd variables ==
  In1 : Inport  OutDataType=sfix(16)  OutScaling=2^0
  Bus Selector5 : BusSelector  OutputSignals=rate.cvc,att.cvc,vel.cvc,pos.cvc
  Demux1 : Demux  Outputs=3
  Demux2 : Demux
  Demux3 : Demux  Outputs=3
  Demux4 : Demux  Outputs=3
  Mux : Mux  Inputs=13
  Subsystem : Subsystem  TreatAsAtomicUnit=on
      settings: RTWSystemCode=Inline
  Out1 : Outport  OutDataType=sfix(16)  OutScaling=2^0
  wires:
  Subsystem/1(Out1) -> Mux/1  "CLAW_p_cvcmd"
  Subsystem/2(Out2) -> Mux/2  "CLAW_q_cvcmd"
  Subsystem/3(Out3) -> Mux/3  "CLAW_r_cvcmd"
  Subsystem/4(Out4) -> Mux/4  "CLAW_e0_cvcmd"
  Subsystem/5(Out5) -> Mux/5  "CLAW_e1_cvcmd"
  Subsystem/6(Out6) -> Mux/6  "CLAW_e2_cvcmd"
  Subsystem/8(Out8) -> Mux/8  "CLAW_Ndot_cvcmd"
  Subsystem/9(Out9) -> Mux/9  "CLAW_Edot_cvcmd"
  Subsystem/10(Out10) -> Mux/10  "CLAW_hdot_cvcmd"
  Subsystem/11(Out11) -> Mux/11  "CLAW_N_cvcmd"
  Subsystem/12(Out12) -> Mux/12  "CLAW_E_cvcmd"
  Subsystem/13(Out13) -> Mux/13  "CLAW_h_cvcmd"
  Subsystem/7(Out7) -> Mux/7  "CLAW_e3_cvcmd"
  In1/1 -> Bus Selector5/1
  Mux/1 -> Out1/1
  Demux1/1 -> Subsystem/1(In1)
  Demux1/2 -> Subsystem/2(In2)
  Demux1/3 -> Subsystem/3(In3)
  Demux2/1 -> Subsystem/4(In4)
  Demux2/2 -> Subsystem/5(In5)
  Demux2/3 -> Subsystem/6(In6)
  Demux2/4 -> Subsystem/7(In7)
  Demux3/1 -> Subsystem/8(In8)
  Demux3/2 -> Subsystem/9(In9)
  Demux3/3 -> Subsystem/10(In10)
  Demux4/1 -> Subsystem/11(In11)
  Demux4/2 -> Subsystem/12(In12)
  Demux4/3 -> Subsystem/13(In13)
  Bus Selector5/4 -> Demux4/1  "<cvc>"
  Bus Selector5/2 -> Demux2/1  "<cvc>"
  Bus Selector5/1 -> Demux1/1  "<cvc>"
  Bus Selector5/3 -> Demux3/1  "<cvc>"

== system main_sim_adapt_Gref_SP/claw_main/grab ExportedGlobal/grab cvdex variables ==
  In1 : Inport  OutDataType=sfix(16)  OutScaling=2^0
  Bus Selector3 : BusSelector  OutputSignals=rate.cvdex,att.cvdex,vel.cvdex,pos.cvdex
  Demux1 : Demux  Outputs=3
  Demux2 : Demux
  Demux3 : Demux  Outputs=3
  Demux4 : Demux  Outputs=3
  Mux : Mux  Inputs=13
  Subsystem : Subsystem  TreatAsAtomicUnit=on
      settings: RTWSystemCode=Inline
  Out1 : Outport  OutDataType=sfix(16)  OutScaling=2^0
  wires:
  Subsystem/1(Out1) -> Mux/1  "CLAW_p_cvdex"
  Subsystem/2(Out2) -> Mux/2  "CLAW_q_cvdex"
  Subsystem/3(Out3) -> Mux/3  "CLAW_r_cvdex"
  Subsystem/4(Out4) -> Mux/4  "CLAW_e0_cvdex"
  Subsystem/5(Out5) -> Mux/5  "CLAW_e1_cvdex"
  Subsystem/6(Out6) -> Mux/6  "CLAW_e2_cvdex"
  Subsystem/8(Out8) -> Mux/8  "CLAW_Ndot_cvdex"
  Subsystem/9(Out9) -> Mux/9  "CLAW_Edot_cvdex"
  Subsystem/10(Out10) -> Mux/10  "CLAW_hdot_cvdex"
  Subsystem/11(Out11) -> Mux/11  "CLAW_N_cvdex"
  Subsystem/12(Out12) -> Mux/12  "CLAW_E_cvdex"
  Subsystem/13(Out13) -> Mux/13  "CLAW_h_cvdex"
  Subsystem/7(Out7) -> Mux/7  "CLAW_e3_cvdex"
  Demux1/1 -> Subsystem/1(In1)
  Demux1/2 -> Subsystem/2(In2)
  Demux1/3 -> Subsystem/3(In3)
  Demux2/1 -> Subsystem/4(In4)
  Demux2/2 -> Subsystem/5(In5)
  Demux2/3 -> Subsystem/6(In6)
  Demux2/4 -> Subsystem/7(In7)
  Demux3/1 -> Subsystem/8(In8)
  Demux3/2 -> Subsystem/9(In9)
  Demux3/3 -> Subsystem/10(In10)
  Demux4/1 -> Subsystem/11(In11)
  Demux4/2 -> Subsystem/12(In12)
  Demux4/3 -> Subsystem/13(In13)
  Mux/1 -> Out1/1
  In1/1 -> Bus Selector3/1
  Bus Selector3/4 -> Demux4/1  "<cvdex>"
  Bus Selector3/3 -> Demux3/1  "<cvdex>"
  Bus Selector3/2 -> Demux2/1  "<cvdex>"
  Bus Selector3/1 -> Demux1/1  "<cvdex>"

== system main_sim_adapt_Gref_SP/claw_main/grab ExportedGlobal/grab integrator variables ==
  In1 : Inport  OutDataType=sfix(16)  OutScaling=2^0
  Bus Selector4 : BusSelector  OutputSignals=rate.integ,att.integ,vel.integ,pos.integ
  Demux1 : Demux  Outputs=3
  Demux2 : Demux
  Demux3 : Demux  Outputs=3
  Demux4 : Demux  Outputs=3
  Mux : Mux  Inputs=13
  Subsystem : Subsystem  TreatAsAtomicUnit=on
      settings: RTWSystemCode=Inline
  Out1 : Outport  OutDataType=sfix(16)  OutScaling=2^0
  wires:
  Subsystem/1(Out1) -> Mux/1  "CLAW_p_int"
  Subsystem/2(Out2) -> Mux/2  "CLAW_q_int"
  Subsystem/3(Out3) -> Mux/3  "CLAW_r_int"
  Subsystem/4(Out4) -> Mux/4  "CLAW_e0_int"
  Subsystem/5(Out5) -> Mux/5  "CLAW_e1_int"
  Subsystem/6(Out6) -> Mux/6  "CLAW_e2_int"
  Subsystem/8(Out8) -> Mux/8  "CLAW_Ndot_int"
  Subsystem/9(Out9) -> Mux/9  "CLAW_Edot_int"
  Subsystem/10(Out10) -> Mux/10  "CLAW_hdot_int"
  Subsystem/11(Out11) -> Mux/11  "CLAW_N_int"
  Subsystem/12(Out12) -> Mux/12  "CLAW_E_int"
  Subsystem/13(Out13) -> Mux/13  "CLAW_h_int"
  Subsystem/7(Out7) -> Mux/7  "CLAW_e3_int"
  Mux/1 -> Out1/1
  Demux1/1 -> Subsystem/1(In1)
  Demux1/2 -> Subsystem/2(In2)
  Demux1/3 -> Subsystem/3(In3)
  Demux2/1 -> Subsystem/4(In4)
  Demux2/2 -> Subsystem/5(In5)
  Demux2/3 -> Subsystem/6(In6)
  Demux2/4 -> Subsystem/7(In7)
  Demux3/1 -> Subsystem/8(In8)
  Demux3/2 -> Subsystem/9(In9)
  Demux3/3 -> Subsystem/10(In10)
  Demux4/1 -> Subsystem/11(In11)
  Demux4/2 -> Subsystem/12(In12)
  Demux4/3 -> Subsystem/13(In13)
  In1/1 -> Bus Selector4/1
  Bus Selector4/4 -> Demux4/1  "<integ>"
  Bus Selector4/3 -> Demux3/1  "<integ>"
  Bus Selector4/2 -> Demux2/1  "<integ>"
  Bus Selector4/1 -> Demux1/1  "<integ>"

== system main_sim_adapt_Gref_SP/claw_main/grab ExportedGlobal/grab w_est variables ==
  In1 : Inport  OutDataType=sfix(16)  OutScaling=2^0
  Bus Selector12 : BusSelector  OutputSignals=w_est_debug.w_est
  Demux1 : Demux  Outputs=3
  Mux : Mux  Inputs=3
  Subsystem : Subsystem  TreatAsAtomicUnit=on
      settings: RTWSystemCode=Inline
  Out1 : Outport  OutDataType=sfix(16)  OutScaling=2^0
  wires:
  Subsystem/1(Out1) -> Mux/1  "CLAW_Nd_wind"
  Subsystem/2(Out2) -> Mux/2  "CLAW_Ed_wind"
  Subsystem/3(Out3) -> Mux/3  "CLAW_Dd_wind"
  Demux1/1 -> Subsystem/1(In1)
  Demux1/2 -> Subsystem/2(In2)
  Demux1/3 -> Subsystem/3(In3)
  Mux/1 -> Out1/1
  Bus Selector12/1 -> Demux1/1  "<w_est>"
  In1/1 -> Bus Selector12/1

== system main_sim_adapt_Gref_SP/claw_main/input processing/mode dependent stick processing ==
  command : Inport  OutDataType=sfix(16)  OutScaling=2^0
  signal_bus : Inport  Port=2  OutDataType=sfix(16)  OutScaling=2^0
  Bus Creator : BusCreator  Inputs=2
  Bus Selector1 : BusSelector  OutputSignals=control_params.accel_cmd_sw,mode_sw.CLAW_mode
  Bus Selector2 : BusSelector  OutputSignals=y_meas.NEh_dot,x_est
  att rate cmd : Subsystem
  att_type cmd : Subsystem
  feed forward : Subsystem
  llh cmd : Subsystem
  rampin vel_cmd : Subsystem
  set command selection switches : Subsystem
  table iv computation : Subsystem
  use table lookup pos cmds : Subsystem
  cmd_bus : Outport  OutDataType=sfix(16)  OutScaling=2^0
  feed_forward : Outport  Port=2  OutDataType=sfix(16)  OutScaling=2^0
  wires:
  Bus Selector1/2 -> set command selection switches/2(CLAW_mode), att rate cmd/1(mode), llh cmd/1(mode), rampin vel_cmd/1(mode), use table lookup pos cmds/1(mode), att_type cmd/1(mode)  "<CLAW_mode>"
  signal_bus/1 -> Bus Selector1/1, llh cmd/3(signal_bus), att rate cmd/3(signal_bus), Bus Selector2/1, att_type cmd/3(signal_bus), feed forward/2(signal_bus)
  llh cmd/1(command_out) -> att rate cmd/2(command_in)
  Bus Selector2/1 -> rampin vel_cmd/3(NEh_dot)  "<NEh_dot>"
  Bus Selector1/1 -> set command selection switches/1(accel_cmd_sw)  "<accel_cmd_sw>"
  set command selection switches/1(select_cmd) -> Bus Creator/1  "select_cmd"
  rampin vel_cmd/1(command_out) -> use table lookup pos cmds/2(command_in)
  Bus Creator/1 -> cmd_bus/1
  use table lookup pos cmds/1(command_out) -> Bus Creator/2  "autopilot_cmd"
  Bus Selector2/2 -> table iv computation/1(x_est)  "<x_est>"
  table iv computation/1(table_bus) -> use table lookup pos cmds/3(table_bus), feed forward/1(table_bus)
  feed forward/1(feed_forward) -> feed_forward/1
  command/1 -> llh cmd/2(command_in)
  att_type cmd/1(command_out) -> rampin vel_cmd/2(command_in)
  att rate cmd/1(command_out) -> att_type cmd/2(command_in)
